simulink model "taolun1"  (R2018a)
settings: Solver=VariableStepAuto  StartTime=0.0  StopTime=10  RelTol=1e-3
settings Model: SnapshotBufferSize=1  SnapshotInterval=1  Creator=edward  LastModifiedBy=edward

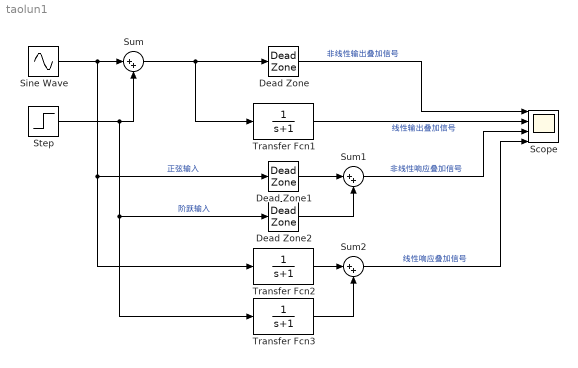
== system taolun1 ==
  Dead Zone : DeadZone  SaturateOnIntegerOverflow=on
  Dead Zone1 : DeadZone  SaturateOnIntegerOverflow=on
  Dead Zone2 : DeadZone  SaturateOnIntegerOverflow=on
  Scope : Scope  NumInputPorts=4
  Sine Wave : Sin  SampleTime=0
  Step : Step  SampleTime=0
  Sum : Sum  Inputs=|++
  Sum1 : Sum  Inputs=|++
  Sum2 : Sum  Inputs=|++
  Transfer Fcn1 : TransferFcn  Denominator=[1 1]
  Transfer Fcn2 : TransferFcn  Denominator=[1 1]
  Transfer Fcn3 : TransferFcn  Denominator=[1 1]
  wires:
  Sine Wave/1 -> Sum/1, Transfer Fcn2/1, Dead Zone1/1  "正弦输入"
  Step/1 -> Transfer Fcn3/1, Dead Zone2/1, Sum/2  "阶跃输入"
  Sum/1 -> Transfer Fcn1/1, Dead Zone/1
  Dead Zone1/1 -> Sum1/1
  Dead Zone2/1 -> Sum1/2
  Sum1/1 -> Scope/3  "非线性响应叠加信号"
  Dead Zone/1 -> Scope/1  "非线性输出叠加信号"
  Transfer Fcn1/1 -> Scope/2  "线性输出叠加信号"
  Transfer Fcn2/1 -> Sum2/1
  Transfer Fcn3/1 -> Sum2/2
  Sum2/1 -> Scope/4  "线性响应叠加信号"
